simulink model "control_project"  (R2018b)
settings: Solver=VariableStepAuto  StartTime=0.0  StopTime=10.0  RelTol=1e-3
settings Model: Creator=Mohammad  LastModifiedBy=Mahdi
settings DataIOCC: ReturnWorkspaceOutputs=on

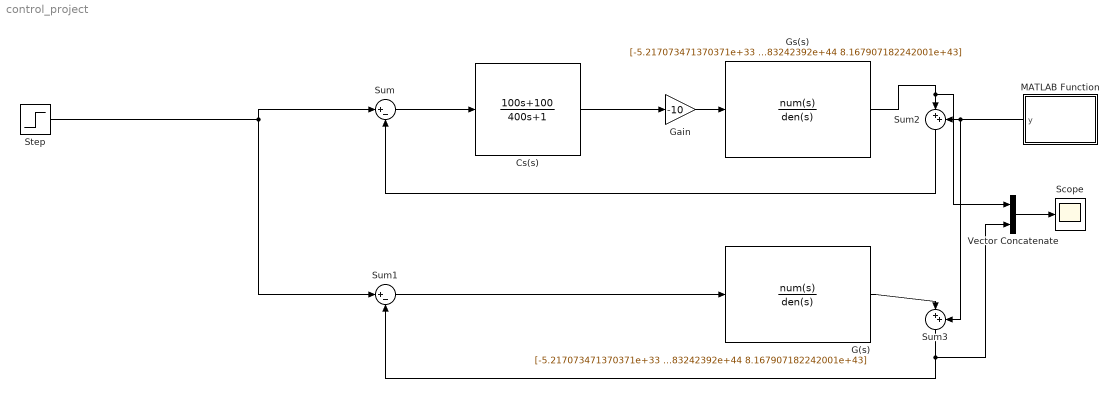
== system control_project ==
  Cs(s) : TransferFcn  Numerator=[100 100]  Denominator=[400 1]
  G(s) : TransferFcn  Numerator=[-5.217073471370371e+33 -2.931768557493656e+36 -6.264908168528483e+38 -6.152454710263484e+40 -2.553422156367967e+42 -2.586887670160663e+43 -1.229374040639164e+44 -3.278043827830406e+44 -5.202909446585797e+44 -4.889150259574264e+44 -2.514965209123656e+44 -5.463736469354852e+43]  Denominator=[1.086630022845231e+33 6.158559214938533e+35 1.337790896719903e+38 1.359305059515519e+40 6.153753385650945e+41 9.116405672458006e+42 6.384944167537608e+43 2.509075291340627e+44 5.965765090188387e+44 8.779009544830330e+44 7.823843860450547e+44 3.871557783242392e+44 8.167907182242001e+43]
  Gain : Gain  Gain=-10
  Gs(s) : TransferFcn  Numerator=[-5.217073471370371e+33 -2.931768557493656e+36 -6.264908168528483e+38 -6.152454710263484e+40 -2.553422156367967e+42 -2.586887670160663e+43 -1.229374040639164e+44 -3.278043827830406e+44 -5.202909446585797e+44 -4.889150259574264e+44 -2.514965209123656e+44 -5.463736469354852e+43]  Denominator=[1.086630022845231e+33 6.158559214938533e+35 1.337790896719903e+38 1.359305059515519e+40 6.153753385650945e+41 9.116405672458006e+42 6.384944167537608e+43 2.509075291340627e+44 5.965765090188387e+44 8.779009544830330e+44 7.823843860450547e+44 3.871557783242392e+44 8.167907182242001e+43]
  MATLAB Function : MATLAB Function  TreatAsAtomicUnit=on
  Scope : Scope
  Step : Step  SampleTime=0
  Sum : Sum  Inputs=|+-
  Sum1 : Sum  Inputs=|+-
  Sum2 : Sum  Inputs=|++
  Sum3 : Sum  Inputs=|++
  Vector Concatenate : Concatenate
  wires:
  Cs(s)/1 -> Gain/1
  Vector Concatenate/1 -> Scope/1
  Gain/1 -> Gs(s)/1
  Sum/1 -> Cs(s)/1
  Sum1/1 -> G(s)/1
  Step/1 -> Sum1/1, Sum/1
  Gs(s)/1 -> Vector Concatenate/1, Sum2/1
  Sum2/1 -> Sum/2
  MATLAB Function/1(y) -> Sum3/2, Sum2/2
  G(s)/1 -> Sum3/1
  Sum3/1 -> Vector Concatenate/2, Sum1/2

== matlab function control_project/MATLAB Function ==
  data: y output
function y = fcn()
y =0.01*randn;
